simulink model "motion_generator"  (R2014b)
settings: Solver=ode3  StartTime=0.0  StopTime=simtime  FixedStep=0.01  RelTol=1e-3
values from neighbouring files (symbols this model uses):
  init_theta = pi    (= 3.14159265359)    [motion_planner.m]
  init_theta_d = -12    [motion_planner.m]
  motion_parameters = [-20 0.3 3]    [motion_planner.m]    (also in path_config.m = [3 0.3]; run_visual.m = [a c w])
settings Model: Creator=Fredrik  LastModifiedBy=Fredrik

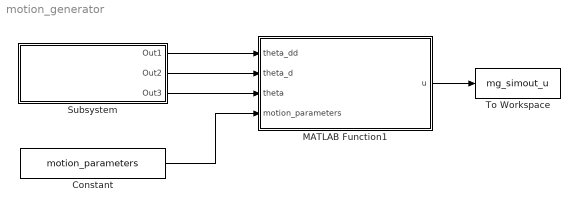
== system motion_generator ==
  Constant : Constant  Value=motion_parameters
  MATLAB Function1 : MATLAB Function  TreatAsAtomicUnit=on
  Subsystem : Subsystem
  To Workspace : ToWorkspace  VariableName=mg_simout_u  SaveFormat=Structure With Time  SampleTime=-1
  wires:
  Subsystem/1(Out1) -> MATLAB Function1/1(theta_dd)
  Subsystem/2(Out2) -> MATLAB Function1/2(theta_d)
  Subsystem/3(Out3) -> MATLAB Function1/3(theta)
  Constant/1 -> MATLAB Function1/4(motion_parameters)
  MATLAB Function1/1(u) -> To Workspace/1

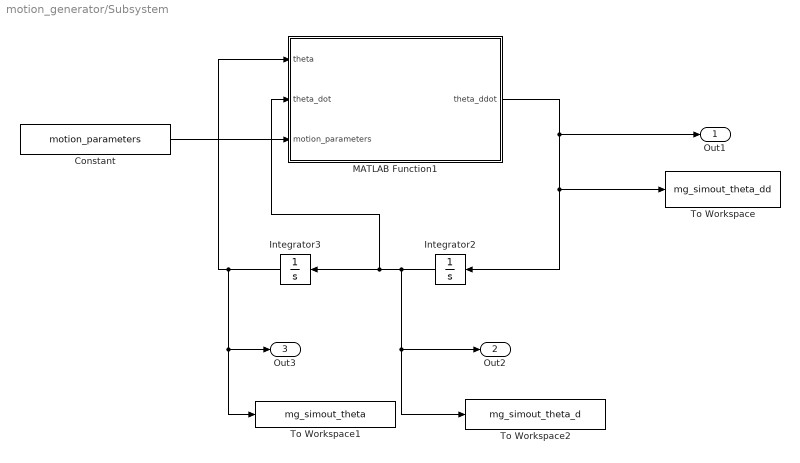
== system motion_generator/Subsystem ==
  Constant : Constant  Value=motion_parameters
  Integrator2 : Integrator  InitialCondition=init_theta_d
  Integrator3 : Integrator  InitialCondition=init_theta
  MATLAB Function1 : MATLAB Function  TreatAsAtomicUnit=on
  To Workspace : ToWorkspace  VariableName=mg_simout_theta_dd  SaveFormat=Structure With Time  SampleTime=-1
  To Workspace1 : ToWorkspace  VariableName=mg_simout_theta  SaveFormat=Structure With Time  SampleTime=-1
  To Workspace2 : ToWorkspace  VariableName=mg_simout_theta_d  SaveFormat=Structure With Time  SampleTime=-1
  Out1 : Outport
  Out2 : Outport  Port=2
  Out3 : Outport  Port=3
  wires:
  MATLAB Function1/1(theta_ddot) -> Out1/1, To Workspace/1, Integrator2/1
  Constant/1 -> MATLAB Function1/3(motion_parameters)
  Integrator2/1 -> Out2/1, To Workspace2/1, Integrator3/1, MATLAB Function1/2(theta_dot)
  Integrator3/1 -> Out3/1, To Workspace1/1, MATLAB Function1/1(theta)

== matlab function motion_generator/Subsystem/MATLAB Function1 ==
  data: theta input; theta_ddot output; theta_dot input; motion_parameters input
function theta_ddot  = fcn(theta, theta_dot, motion_parameters)
%#codegen

g=9.81;

a=motion_parameters(1);
c=motion_parameters(2);
w=motion_parameters(3);

alfa=cos(theta)*(-cos(theta)*c*w+1)/w+1;
beta=cos(theta)*c*sin(theta);
gamma=-2*cos(theta)*a/w-g*sin(theta);




theta_ddot = (-beta*(theta_dot^2) - gamma)/alfa;

== matlab function motion_generator/MATLAB Function1 ==
  data: theta_dd input; theta_d input; u output; theta input; motion_parameters input
function u = fcn(theta_dd, theta_d, theta,motion_parameters)

a=motion_parameters(1)
c=motion_parameters(2);
w=motion_parameters(3);


u=((2*(-cos(theta)*c*w+1))/w+cos(theta))*(theta_dd)+(2*c*sin(theta)-sin(theta))*(theta_d)^2-4*a/w;
